simulink model "HC_core_compensation_all"  (R2023b)
settings: configuration reference "slow_tsk_conf" (kept outside this file)
undefined symbols (not defined in the file): shuntNumHarmonics
settings Model: DataDictionary=fmuGenerationDictionay.sldd  Creator=Veimar  LastModifiedBy=Veimar
settings ConfigSetRef: SourceName=slow_tsk_conf

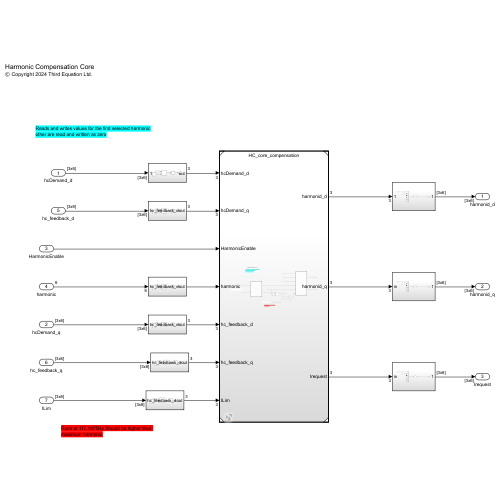
[thumbnail: Simulink's stored preview of the top-level diagram]
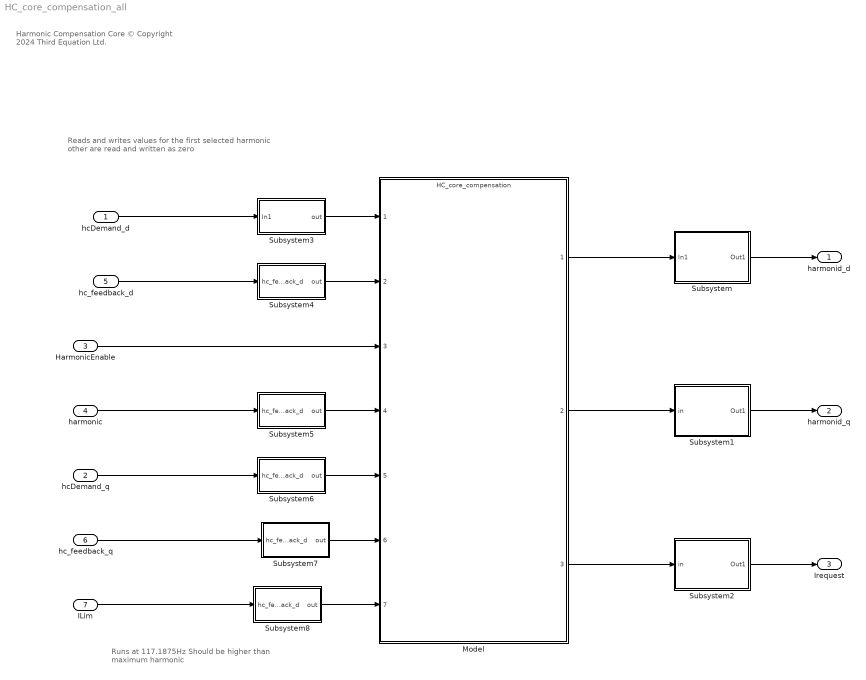
== system HC_core_compensation_all ==
  note: Reads and writes values for the first selected harmonic
      | other are read and written as zero
  note: Harmonic Compensation Core
      | © Copyright 2024 Third Equation Ltd.
  note: Runs at 117.1875Hz Should be higher than
      | maximum harmonic
  hcDemand_d : Inport  OutDataTypeStr=single  PortDimensions=[3 shuntNumHarmonics]
  hcDemand_q : Inport  Port=2  OutDataTypeStr=single  PortDimensions=[3 shuntNumHarmonics]
  HarmonicEnable : Inport  Port=3  OutDataTypeStr=boolean  PortDimensions=1
  harmonic : Inport  Port=4  OutDataTypeStr=single  PortDimensions=shuntNumHarmonics
  hc_feedback_d : Inport  Port=5  OutDataTypeStr=single  PortDimensions=[3 shuntNumHarmonics]
  hc_feedback_q : Inport  Port=6  OutDataTypeStr=single  PortDimensions=[3 shuntNumHarmonics]
  ILim : Inport  Port=7  OutDataTypeStr=single  PortDimensions=[3 shuntNumHarmonics]
  Model : ModelReference  ModelNameDialog=HC_core_compensation.slx  SimulationMode=Normal  ModelReferenceVersion=1.32
  Subsystem : Subsystem
  Subsystem1 : Subsystem
  Subsystem2 : Subsystem
  Subsystem3 : Subsystem
  Subsystem4 : Subsystem
  Subsystem5 : Subsystem
  Subsystem6 : Subsystem
  Subsystem7 : Subsystem
  Subsystem8 : Subsystem
  harmonid_d : Outport  OutDataTypeStr=single  PortDimensions=[3 shuntNumHarmonics]
  harmonid_q : Outport  Port=2  OutDataTypeStr=single  PortDimensions=[3 shuntNumHarmonics]
  Irequest : Outport  Port=3  OutDataTypeStr=single  PortDimensions=[3 shuntNumHarmonics]
  wires:
  hcDemand_d/1 -> Subsystem3/1(In1)
  hcDemand_q/1 -> Subsystem6/1(hc_feedback_d)
  Subsystem1/1(Out1) -> harmonid_q/1
  HarmonicEnable/1 -> Model/3
  hc_feedback_d/1 -> Subsystem4/1(hc_feedback_d)
  hc_feedback_q/1 -> Subsystem7/1(hc_feedback_d)
  harmonic/1 -> Subsystem5/1(hc_feedback_d)
  ILim/1 -> Subsystem8/1(hc_feedback_d)
  Subsystem2/1(Out1) -> Irequest/1
  Model/1 -> Subsystem/1(In1)
  Subsystem/1(Out1) -> harmonid_d/1
  Model/2 -> Subsystem1/1(in)
  Model/3 -> Subsystem2/1(in)
  Subsystem3/1(out) -> Model/1
  Subsystem4/1(out) -> Model/2
  Subsystem5/1(out) -> Model/4
  Subsystem6/1(out) -> Model/5
  Subsystem7/1(out) -> Model/6
  Subsystem8/1(out) -> Model/7

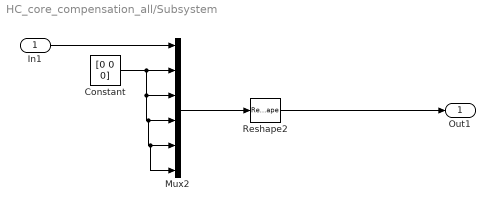
== system HC_core_compensation_all/Subsystem ==
  In1 : Inport
  Constant : Constant  Value=[0 0 0]  OutDataTypeStr=single
  Mux2 : Mux  Inputs=6
  Reshape2 : Reshape  OutputDimensionality=Customize  OutputDimensions=[3,6]
  Out1 : Outport
  wires:
  Mux2/1 -> Reshape2/1
  Constant/1 -> Mux2/6, Mux2/5, Mux2/4, Mux2/3, Mux2/2
  In1/1 -> Mux2/1
  Reshape2/1 -> Out1/1

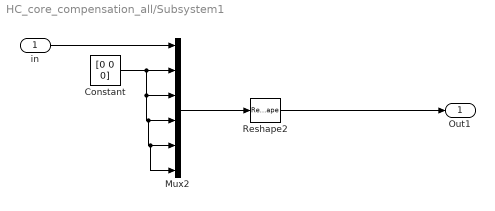
== system HC_core_compensation_all/Subsystem1 ==
  in : Inport
  Constant : Constant  Value=[0 0 0]  OutDataTypeStr=single
  Mux2 : Mux  Inputs=6
  Reshape2 : Reshape  OutputDimensionality=Customize  OutputDimensions=[3,6]
  Out1 : Outport
  wires:
  Reshape2/1 -> Out1/1
  in/1 -> Mux2/1
  Constant/1 -> Mux2/2, Mux2/3, Mux2/4, Mux2/5, Mux2/6
  Mux2/1 -> Reshape2/1

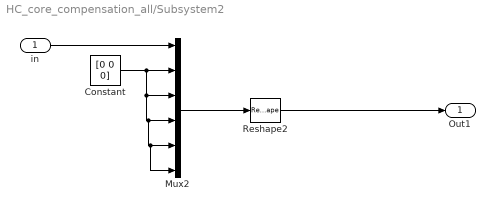
== system HC_core_compensation_all/Subsystem2 ==
  in : Inport
  Constant : Constant  Value=[0 0 0]  OutDataTypeStr=single
  Mux2 : Mux  Inputs=6
  Reshape2 : Reshape  OutputDimensionality=Customize  OutputDimensions=[3,6]
  Out1 : Outport
  wires:
  Mux2/1 -> Reshape2/1
  Constant/1 -> Mux2/6, Mux2/5, Mux2/4, Mux2/3, Mux2/2
  in/1 -> Mux2/1
  Reshape2/1 -> Out1/1

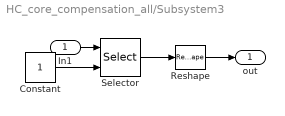
== system HC_core_compensation_all/Subsystem3 ==
  In1 : Inport
  Constant : Constant
  Reshape : Reshape
  Selector : Selector  NumberOfDimensions=2  InputPortWidth=1  IndexOptions=Select all,Index vector (port)  Indices=[1 3],1  OutputSizes=1,1
  out : Outport
  wires:
  Constant/1 -> Selector/2
  Selector/1 -> Reshape/1
  Reshape/1 -> out/1
  In1/1 -> Selector/1

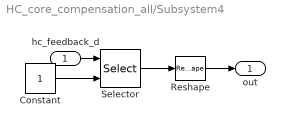
== system HC_core_compensation_all/Subsystem4 ==
  hc_feedback_d : Inport
  Constant : Constant
  Reshape : Reshape
  Selector : Selector  NumberOfDimensions=2  InputPortWidth=1  IndexOptions=Select all,Index vector (port)  Indices=[1 3],1  OutputSizes=1,1
  out : Outport
  wires:
  hc_feedback_d/1 -> Selector/1
  Reshape/1 -> out/1
  Selector/1 -> Reshape/1
  Constant/1 -> Selector/2

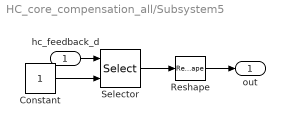
== system HC_core_compensation_all/Subsystem5 ==
  hc_feedback_d : Inport
  Constant : Constant
  Reshape : Reshape
  Selector : Selector  NumberOfDimensions=2  InputPortWidth=1  IndexOptions=Select all,Index vector (port)  Indices=[1 3],1  OutputSizes=1,1
  out : Outport
  wires:
  Constant/1 -> Selector/2
  Selector/1 -> Reshape/1
  Reshape/1 -> out/1
  hc_feedback_d/1 -> Selector/1

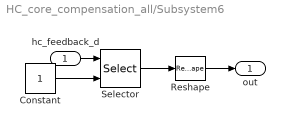
== system HC_core_compensation_all/Subsystem6 ==
  hc_feedback_d : Inport
  Constant : Constant
  Reshape : Reshape
  Selector : Selector  NumberOfDimensions=2  InputPortWidth=1  IndexOptions=Select all,Index vector (port)  Indices=[1 3],1  OutputSizes=1,1
  out : Outport
  wires:
  hc_feedback_d/1 -> Selector/1
  Reshape/1 -> out/1
  Selector/1 -> Reshape/1
  Constant/1 -> Selector/2

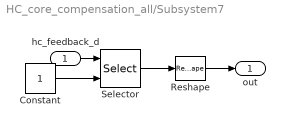
== system HC_core_compensation_all/Subsystem7 ==
  hc_feedback_d : Inport
  Constant : Constant
  Reshape : Reshape
  Selector : Selector  NumberOfDimensions=2  InputPortWidth=1  IndexOptions=Select all,Index vector (port)  Indices=[1 3],1  OutputSizes=1,1
  out : Outport
  wires:
  Constant/1 -> Selector/2
  Selector/1 -> Reshape/1
  Reshape/1 -> out/1
  hc_feedback_d/1 -> Selector/1

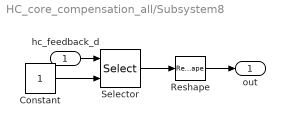
== system HC_core_compensation_all/Subsystem8 ==
  hc_feedback_d : Inport
  Constant : Constant
  Reshape : Reshape
  Selector : Selector  NumberOfDimensions=2  InputPortWidth=1  IndexOptions=Select all,Index vector (port)  Indices=[1 3],1  OutputSizes=1,1
  out : Outport
  wires:
  hc_feedback_d/1 -> Selector/1
  Reshape/1 -> out/1
  Selector/1 -> Reshape/1
  Constant/1 -> Selector/2
